simulink model "modl3"  (Simulink 4.00)
settings: Solver=ode45  StartTime=0.0  StopTime=2.0  RelTol=1e-3
libraries: simulink_extras x1
settings Model: BlockReductionOpt=off

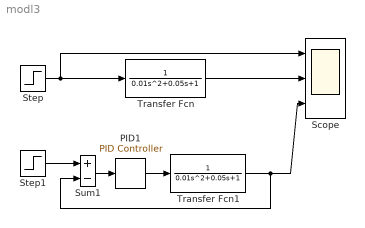
== system modl3 ==
  PID1 : simulink_extras/Additional Linear/PID Controller  P=0.225  I=4.5  D=0.045
  Scope : Scope  NumInputPorts=3
      settings: TimeRange=auto  YMin=-5~-5~-5  YMax=5~5~5  SaveToWorkspace=off  SaveName=ScopeData  MaxDataPoints=5000
  Step : Step  Time=0.1  Before=0  After=1  SampleTime=0
  Step1 : Step  Time=0.1  Before=0  After=1  SampleTime=0
  Sum1 : Sum  Inputs=+-  SaturateOnIntegerOverflow=on
  Transfer Fcn : TransferFcn  Numerator=[1]  Denominator=[0.01 0.05 1]  Realization=auto  AbsoluteTolerance=auto
  Transfer Fcn1 : TransferFcn  Numerator=[1]  Denominator=[0.01 0.05 1]  Realization=auto  AbsoluteTolerance=auto
  wires:
  Step/1 -> Scope/1, Transfer Fcn/1
  Transfer Fcn/1 -> Scope/2
  Sum1/1 -> PID1/1
  PID1/1 -> Transfer Fcn1/1
  Step1/1 -> Sum1/1
  Transfer Fcn1/1 -> Sum1/2, Scope/3
